simulink model "Aileron_AFTC"  (Simulink 8.6)
settings: Solver=FixedStepAuto  StartTime=0.0  StopTime=40  FixedStep=0.01  RelTol=1e-3
libraries: fuzblock x4, simulink x2
settings Model: Creator=Alireza  LastModifiedBy=aabba014
settings SolverCC: ZeroCrossAlgorithm=Adaptive
settings DebuggingCC: FcnCallInpInsideContextMsg=UseLocalSettings

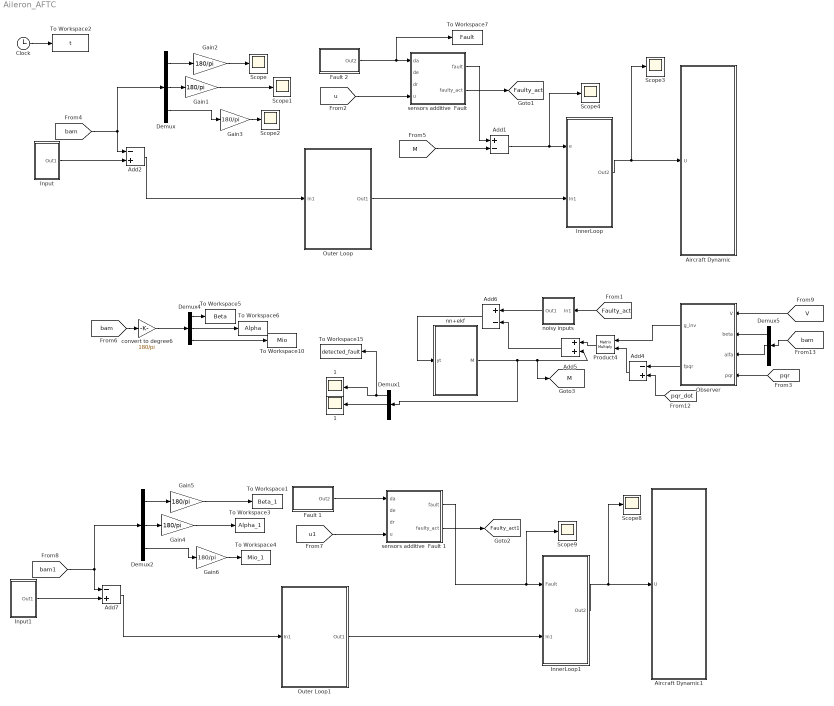
== system Aileron_AFTC ==
  "      1" : Scope
  "     1" : Scope
  Add1 : Sum  Inputs=+-
  Add2 : Sum  Inputs=-+
  Add4 : Sum  Inputs=-+
  Add5 : Sum
  Add6 : Sum  Inputs=+-  OutDataTypeStr=Inherit: Same as accumulator
  Add7 : Sum  Inputs=-+
  Aircraft Dynamic : Subsystem
  Aircraft Dynamic1 : Subsystem
  Clock : Clock
  Demux{,1..2,4..5} (5 alike) : Demux  Outputs=3
  Fault 1 : Subsystem
  Fault 2 : Subsystem
  Gain{1..6} (6 alike) : Gain  Gain=180/pi
  InnerLoop : Subsystem
  InnerLoop1 : Subsystem
  Input : Subsystem
  Input1 : Subsystem
  Observer : MATLAB Function  TreatAsAtomicUnit=on
  Outer Loop : Subsystem
  Outer Loop1 : Subsystem
  Product4 : Product  Multiplication=Matrix(*)  RndMeth=Zero
  Scope{,1..4,8..9} (7 alike) : Scope
  To Workspace1 : ToWorkspace  VariableName=Beta_1  SampleTime=-1
  To Workspace10 : ToWorkspace  VariableName=Mio  SampleTime=-1
  To Workspace15 : ToWorkspace  VariableName=detected_fault  SampleTime=-1
  To Workspace2 : ToWorkspace  VariableName=t  SampleTime=-1
  To Workspace3 : ToWorkspace  VariableName=Alpha_1  SampleTime=-1
  To Workspace4 : ToWorkspace  VariableName=Mio_1  SampleTime=-1
  To Workspace5 : ToWorkspace  VariableName=Beta  SampleTime=-1
  To Workspace6 : ToWorkspace  VariableName=Alpha  SampleTime=-1
  To Workspace7 : ToWorkspace  VariableName=Fault  SampleTime=-1
  convert to degree6 : Gain  Gain=180/pi
  nn+ekf : Subsystem
  noisy inputs : Subsystem
  "sensors additive  Fault " : MATLAB Function  TreatAsAtomicUnit=on
  sensors additive  Fault 1 : MATLAB Function  TreatAsAtomicUnit=on
  tag scope: Faulty_act1=global, Faulty_act=global, M=global
  wires:
  [bam] -> Add2/1, Demux/1
  Input/1(Out1) -> Add2/2
  Outer Loop/1(Out1) -> InnerLoop/2(In1)
  InnerLoop/1(Out2) -> Scope3/1, Aircraft Dynamic/1(U)
  Add2/1 -> Outer Loop/1(In1)
  Demux/1 -> Gain2/1
  Demux/2 -> Gain1/1
  Demux/3 -> Gain3/1
  Gain2/1 -> Scope/1
  Gain1/1 -> Scope1/1
  Gain3/1 -> Scope2/1
  [u] -> "sensors additive  Fault "/4(u)
  "sensors additive  Fault "/2(faulty_act) -> [Faulty_act]
  Add1/1 -> InnerLoop/1(e), Scope4/1
  "sensors additive  Fault "/1(fault) -> Add1/1
  Clock/1 -> To Workspace2/1
  Add5/1 -> Add6/2
  Add6/1 -> nn+ekf/1(yt)
  [bam] -> convert to degree6/1
  [V] -> Observer/1(V)
  [bam] -> Demux5/1
  nn+ekf/1(M) -> Add5/2, [M], Demux1/1
  Demux1/1 -> "     1"/1, To Workspace15/1
  Demux1/2 -> "      1"/1
  convert to degree6/1 -> Demux4/1
  [Faulty_act] -> noisy inputs/1(In1)
  Demux4/1 -> To Workspace5/1
  Demux4/2 -> To Workspace6/1
  Demux4/3 -> To Workspace10/1
  Demux5/1 -> Observer/2(beta)
  Demux5/2 -> Observer/3(alfa)
  [pqr] -> Observer/4(pqr)
  Observer/2(fpqr) -> Add4/1
  [pqr_dot] -> Add4/2
  Add4/1 -> Product4/2
  Observer/1(g_inv) -> Product4/1
  Product4/1 -> Add5/1
  noisy inputs/1(Out1) -> Add6/1
  [M] -> Add1/2
  [bam1] -> Add7/1, Demux2/1
  Input1/1(Out1) -> Add7/2
  Outer Loop1/1(Out1) -> InnerLoop1/2(In1)
  InnerLoop1/1(Out2) -> Aircraft Dynamic1/1(U), Scope8/1
  Add7/1 -> Outer Loop1/1(In1)
  Demux2/1 -> Gain5/1
  Demux2/2 -> Gain4/1
  Demux2/3 -> Gain6/1
  Gain5/1 -> To Workspace1/1
  Gain4/1 -> To Workspace3/1
  [u1] -> sensors additive  Fault 1/4(u)
  sensors additive  Fault 1/2(faulty_act) -> [Faulty_act1]
  sensors additive  Fault 1/1(fault) -> InnerLoop1/1(Fault), Scope9/1
  Gain6/1 -> To Workspace4/1
  Fault 2/1(Out2) -> "sensors additive  Fault "/1(da), To Workspace7/1
  Fault 1/1(Out2) -> sensors additive  Fault 1/1(da)

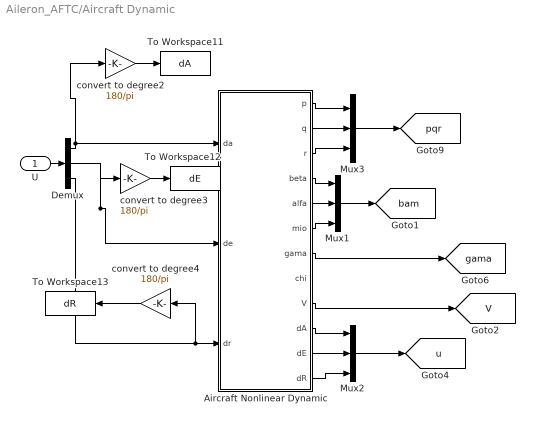
== system Aileron_AFTC/Aircraft Dynamic ==
  U : Inport
  Aircraft Nonlinear Dynamic : Subsystem
  Demux : Demux  Outputs=3
  Mux1 : Mux  Inputs=3
  Mux2 : Mux  Inputs=3
  Mux3 : Mux  Inputs=3
  To Workspace11 : ToWorkspace  VariableName=dA  SampleTime=-1
  To Workspace12 : ToWorkspace  VariableName=dE  SampleTime=-1
  To Workspace13 : ToWorkspace  VariableName=dR  SampleTime=-1
  convert to degree2 : Gain  Gain=180/pi
  convert to degree3 : Gain  Gain=180/pi
  convert to degree4 : Gain  Gain=180/pi
  tag scope: V=global, bam=global, gama=global, pqr=global, u=global
  wires:
  Aircraft Nonlinear Dynamic/4(beta) -> Mux1/1
  Aircraft Nonlinear Dynamic/5(alfa) -> Mux1/2
  Aircraft Nonlinear Dynamic/6(mio) -> Mux1/3
  Mux1/1 -> [bam]
  Aircraft Nonlinear Dynamic/9(V) -> [V]
  Aircraft Nonlinear Dynamic/7(gama) -> [gama]
  Aircraft Nonlinear Dynamic/1(p) -> Mux3/1
  Aircraft Nonlinear Dynamic/2(q) -> Mux3/2
  Aircraft Nonlinear Dynamic/3(r) -> Mux3/3
  Mux3/1 -> [pqr]
  Aircraft Nonlinear Dynamic/10(dA) -> Mux2/1
  Aircraft Nonlinear Dynamic/11(dE) -> Mux2/2
  Aircraft Nonlinear Dynamic/12(dR) -> Mux2/3
  Mux2/1 -> [u]
  convert to degree2/1 -> To Workspace11/1
  convert to degree3/1 -> To Workspace12/1
  Demux/2 -> convert to degree3/1, Aircraft Nonlinear Dynamic/2(de)
  Demux/3 -> Aircraft Nonlinear Dynamic/3(dr), convert to degree4/1
  convert to degree4/1 -> To Workspace13/1
  U/1 -> Demux/1
  Demux/1 -> convert to degree2/1, Aircraft Nonlinear Dynamic/1(da)

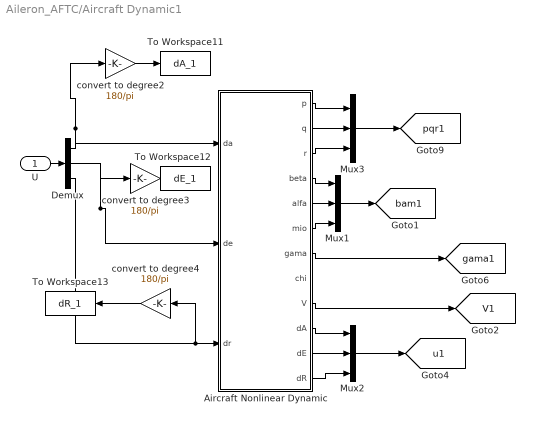
== system Aileron_AFTC/Aircraft Dynamic1 ==
  U : Inport
  Aircraft Nonlinear Dynamic : Subsystem
  Demux : Demux  Outputs=3
  Mux1 : Mux  Inputs=3
  Mux2 : Mux  Inputs=3
  Mux3 : Mux  Inputs=3
  To Workspace11 : ToWorkspace  VariableName=dA_1  SampleTime=-1
  To Workspace12 : ToWorkspace  VariableName=dE_1  SampleTime=-1
  To Workspace13 : ToWorkspace  VariableName=dR_1  SampleTime=-1
  convert to degree2 : Gain  Gain=180/pi
  convert to degree3 : Gain  Gain=180/pi
  convert to degree4 : Gain  Gain=180/pi
  tag scope: V1=global, bam1=global, gama1=global, pqr1=global, u1=global
  wires:
  Aircraft Nonlinear Dynamic/4(beta) -> Mux1/1
  Aircraft Nonlinear Dynamic/5(alfa) -> Mux1/2
  Aircraft Nonlinear Dynamic/6(mio) -> Mux1/3
  Mux1/1 -> [bam1]
  Aircraft Nonlinear Dynamic/9(V) -> [V1]
  Aircraft Nonlinear Dynamic/7(gama) -> [gama1]
  Aircraft Nonlinear Dynamic/1(p) -> Mux3/1
  Aircraft Nonlinear Dynamic/2(q) -> Mux3/2
  Aircraft Nonlinear Dynamic/3(r) -> Mux3/3
  Mux3/1 -> [pqr1]
  Aircraft Nonlinear Dynamic/10(dA) -> Mux2/1
  Aircraft Nonlinear Dynamic/11(dE) -> Mux2/2
  Aircraft Nonlinear Dynamic/12(dR) -> Mux2/3
  Mux2/1 -> [u1]
  convert to degree2/1 -> To Workspace11/1
  convert to degree3/1 -> To Workspace12/1
  Demux/2 -> convert to degree3/1, Aircraft Nonlinear Dynamic/2(de)
  Demux/3 -> Aircraft Nonlinear Dynamic/3(dr), convert to degree4/1
  convert to degree4/1 -> To Workspace13/1
  U/1 -> Demux/1
  Demux/1 -> convert to degree2/1, Aircraft Nonlinear Dynamic/1(da)

== system Aileron_AFTC/Fault 1 ==
  Add13 : Sum  Inputs=+-
  Ramp : simulink/Sources/Ramp  slope=1  start=0  X0=0
  Triangular MF : fuzblock/Membership  Functions/Triangular MF  a=3  b=7  c=11
  Triangular MF1 : fuzblock/Membership  Functions/Triangular MF  a=11  b=15  c=19
  Out2 : Outport
  wires:
  Ramp/1 -> Triangular MF/1, Triangular MF1/1
  Triangular MF/1 -> Add13/1
  Add13/1 -> Out2/1

== system Aileron_AFTC/Fault 2 ==
  Add13 : Sum  Inputs=+-
  Ramp : simulink/Sources/Ramp  slope=1  start=0  X0=0
  Triangular MF : fuzblock/Membership  Functions/Triangular MF  a=3  b=7  c=11
  Triangular MF1 : fuzblock/Membership  Functions/Triangular MF  a=11  b=15  c=19
  Out2 : Outport
  wires:
  Ramp/1 -> Triangular MF/1, Triangular MF1/1
  Triangular MF/1 -> Add13/1
  Add13/1 -> Out2/1

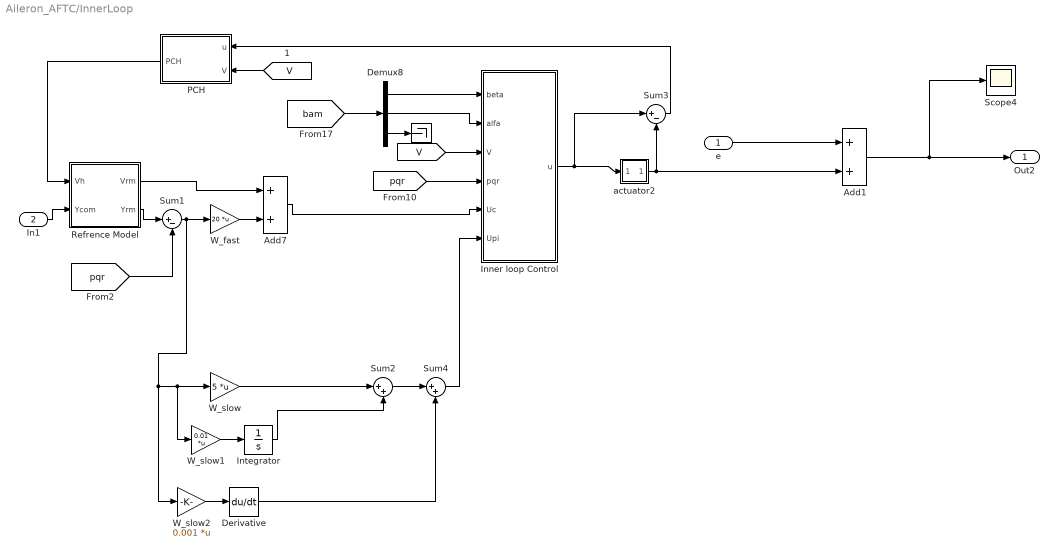
== system Aileron_AFTC/InnerLoop ==
  e : Inport
  In1 : Inport  Port=2
  "  " : Terminator
  Add1 : Sum
  Add7 : Sum
  Demux8 : Demux  Outputs=3
  Derivative : Derivative
  Inner loop Control : MATLAB Function  TreatAsAtomicUnit=on
  Integrator : Integrator
  PCH : MATLAB Function  TreatAsAtomicUnit=on
  Refrence Model : Subsystem
  Scope4 : Scope
  Sum1 : Sum  Inputs=|+-
  Sum2 : Sum  Inputs=|++
  Sum3 : Sum  Inputs=|+-
  Sum4 : Sum  Inputs=|++
  W_fast : Gain  Gain=20  Multiplication=Matrix(K*u)
  W_slow : Gain  Gain=5  Multiplication=Matrix(K*u)
  W_slow1 : Gain  Gain=0.01  Multiplication=Matrix(K*u)
  W_slow2 : Gain  Gain=0.001  Multiplication=Matrix(K*u)
  actuator2 : Subsystem
  Out2 : Outport
  wires:
  [V] -> Inner loop Control/3(V)
  [bam] -> Demux8/1
  Demux8/1 -> Inner loop Control/1(beta)
  Demux8/2 -> Inner loop Control/2(alfa)
  Demux8/3 -> "  "/1
  [pqr] -> Inner loop Control/4(pqr)
  [pqr] -> Sum1/2
  Sum1/1 -> W_fast/1, W_slow1/1, W_slow/1, W_slow2/1
  Add7/1 -> Inner loop Control/5(Uc)
  e/1 -> Add1/1
  [V] -> PCH/2(V)
  W_fast/1 -> Add7/2
  In1/1 -> Refrence Model/2(Ycom)
  Refrence Model/1(Vrm) -> Add7/1
  PCH/1(PCH) -> Refrence Model/1(Vh)
  W_slow/1 -> Sum2/1
  W_slow1/1 -> Integrator/1
  Integrator/1 -> Sum2/2
  Refrence Model/2(Yrm) -> Sum1/1
  W_slow2/1 -> Derivative/1
  Sum2/1 -> Sum4/1
  Derivative/1 -> Sum4/2
  Add1/1 -> Out2/1, Scope4/1
  Inner loop Control/1(u) -> Sum3/1, actuator2/1(In1)
  actuator2/1(Out1) -> Sum3/2, Add1/2
  Sum3/1 -> PCH/1(u)
  Sum4/1 -> Inner loop Control/6(Upi)

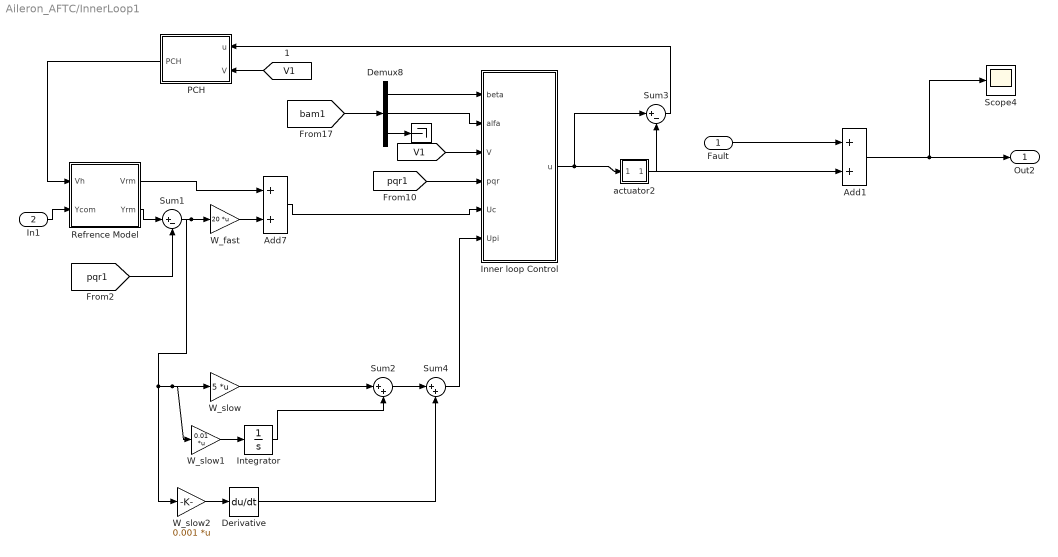
== system Aileron_AFTC/InnerLoop1 ==
  Fault : Inport
  In1 : Inport  Port=2
  "  " : Terminator
  Add1 : Sum
  Add7 : Sum
  Demux8 : Demux  Outputs=3
  Derivative : Derivative
  Inner loop Control : MATLAB Function  TreatAsAtomicUnit=on
  Integrator : Integrator
  PCH : MATLAB Function  TreatAsAtomicUnit=on
  Refrence Model : Subsystem
  Scope4 : Scope
  Sum1 : Sum  Inputs=|+-
  Sum2 : Sum  Inputs=|++
  Sum3 : Sum  Inputs=|+-
  Sum4 : Sum  Inputs=|++
  W_fast : Gain  Gain=20  Multiplication=Matrix(K*u)
  W_slow : Gain  Gain=5  Multiplication=Matrix(K*u)
  W_slow1 : Gain  Gain=0.01  Multiplication=Matrix(K*u)
  W_slow2 : Gain  Gain=0.001  Multiplication=Matrix(K*u)
  actuator2 : Subsystem
  Out2 : Outport
  wires:
  [V1] -> Inner loop Control/3(V)
  [bam1] -> Demux8/1
  Demux8/1 -> Inner loop Control/1(beta)
  Demux8/2 -> Inner loop Control/2(alfa)
  Demux8/3 -> "  "/1
  [pqr1] -> Inner loop Control/4(pqr)
  [pqr1] -> Sum1/2
  Sum1/1 -> W_fast/1, W_slow1/1, W_slow/1, W_slow2/1
  Add7/1 -> Inner loop Control/5(Uc)
  Fault/1 -> Add1/1
  [V1] -> PCH/2(V)
  W_fast/1 -> Add7/2
  In1/1 -> Refrence Model/2(Ycom)
  Refrence Model/1(Vrm) -> Add7/1
  PCH/1(PCH) -> Refrence Model/1(Vh)
  W_slow/1 -> Sum2/1
  W_slow1/1 -> Integrator/1
  Integrator/1 -> Sum2/2
  Refrence Model/2(Yrm) -> Sum1/1
  W_slow2/1 -> Derivative/1
  Sum2/1 -> Sum4/1
  Derivative/1 -> Sum4/2
  Add1/1 -> Out2/1, Scope4/1
  Inner loop Control/1(u) -> Sum3/1, actuator2/1(In1)
  actuator2/1(Out1) -> Sum3/2, Add1/2
  Sum3/1 -> PCH/1(u)
  Sum4/1 -> Inner loop Control/6(Upi)

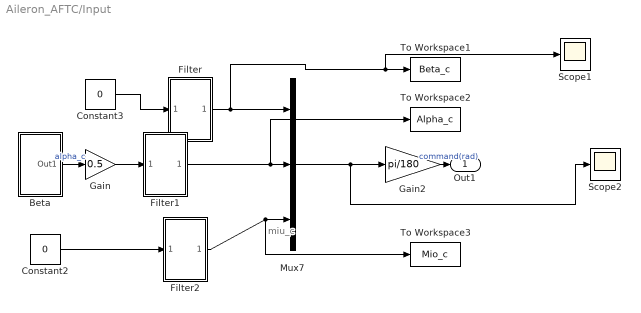
== system Aileron_AFTC/Input ==
  note: miu_c
  Beta : Subsystem
  Constant2 : Constant  Value=0
  Constant3 : Constant  Value=0
  Filter : Subsystem
  Filter1 : Subsystem
  Filter2 : Subsystem
  Gain : Gain  Gain=0.5
  Gain2 : Gain  Gain=pi/180
  Mux7 : Mux  Inputs=3
  Scope1 : Scope
  Scope2 : Scope
  To Workspace1 : ToWorkspace  VariableName=Beta_c  SampleTime=-1
  To Workspace2 : ToWorkspace  VariableName=Alpha_c  SampleTime=-1
  To Workspace3 : ToWorkspace  VariableName=Mio_c  SampleTime=-1
  Out1 : Outport
  wires:
  Beta/1(Out1) -> Gain/1  "alpha_c"
  Constant2/1 -> Filter2/1(In1)
  Mux7/1 -> Gain2/1, Scope2/1
  Gain2/1 -> Out1/1  "command(rad)"
  Filter/1(Out1) -> Mux7/1, To Workspace1/1, Scope1/1
  Filter1/1(Out1) -> Mux7/2, To Workspace2/1
  Filter2/1(Out1) -> Mux7/3, To Workspace3/1
  Constant3/1 -> Filter/1(In1)
  Gain/1 -> Filter1/1(In1)

== system Aileron_AFTC/Input1 ==
  note: miu_c
  Beta : Subsystem
  Constant2 : Constant  Value=0
  Constant3 : Constant  Value=0
  Filter : Subsystem
  Filter1 : Subsystem
  Filter2 : Subsystem
  Gain : Gain  Gain=0.5
  Gain2 : Gain  Gain=pi/180
  Mux7 : Mux  Inputs=3
  Out1 : Outport
  wires:
  Beta/1(Out1) -> Gain/1  "alpha_c"
  Constant2/1 -> Filter2/1(In1)
  Mux7/1 -> Gain2/1
  Gain2/1 -> Out1/1  "command(rad)"
  Filter/1(Out1) -> Mux7/1
  Filter1/1(Out1) -> Mux7/2
  Filter2/1(Out1) -> Mux7/3
  Constant3/1 -> Filter/1(In1)
  Gain/1 -> Filter1/1(In1)

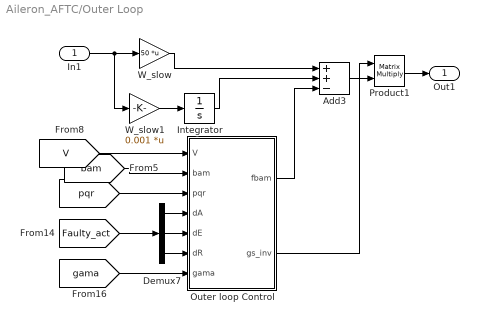
== system Aileron_AFTC/Outer Loop ==
  In1 : Inport
  Add3 : Sum  Inputs=++-
  Demux7 : Demux  Outputs=3
  Integrator : Integrator
  Outer loop Control : MATLAB Function  TreatAsAtomicUnit=on
  Product1 : Product  Multiplication=Matrix(*)  RndMeth=Zero
  W_slow : Gain  Gain=50  Multiplication=Matrix(K*u)
  W_slow1 : Gain  Gain=0.001  Multiplication=Matrix(K*u)
  Out1 : Outport
  wires:
  Outer loop Control/2(gs_inv) -> Product1/1
  Add3/1 -> Product1/2
  [pqr] -> Outer loop Control/3(pqr)
  [bam] -> Outer loop Control/2(bam)
  [V] -> Outer loop Control/1(V)
  [Faulty_act] -> Demux7/1
  Demux7/1 -> Outer loop Control/4(dA)
  Demux7/2 -> Outer loop Control/5(dE)
  Demux7/3 -> Outer loop Control/6(dR)
  [gama] -> Outer loop Control/7(gama)
  In1/1 -> W_slow1/1, W_slow/1
  W_slow/1 -> Add3/1
  W_slow1/1 -> Integrator/1
  Outer loop Control/1(fbam) -> Add3/3
  Integrator/1 -> Add3/2
  Product1/1 -> Out1/1

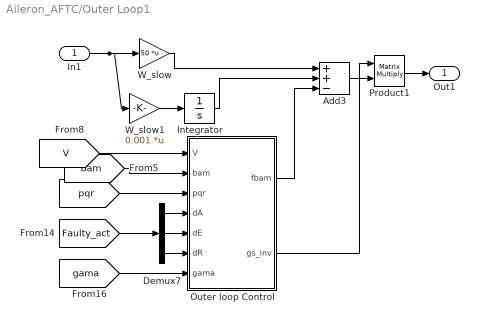
== system Aileron_AFTC/Outer Loop1 ==
  In1 : Inport
  Add3 : Sum  Inputs=++-
  Demux7 : Demux  Outputs=3
  Integrator : Integrator
  Outer loop Control : MATLAB Function  TreatAsAtomicUnit=on
  Product1 : Product  Multiplication=Matrix(*)  RndMeth=Zero
  W_slow : Gain  Gain=50  Multiplication=Matrix(K*u)
  W_slow1 : Gain  Gain=0.001  Multiplication=Matrix(K*u)
  Out1 : Outport
  wires:
  Outer loop Control/2(gs_inv) -> Product1/1
  Add3/1 -> Product1/2
  [pqr] -> Outer loop Control/3(pqr)
  [bam] -> Outer loop Control/2(bam)
  [V] -> Outer loop Control/1(V)
  [Faulty_act] -> Demux7/1
  Demux7/1 -> Outer loop Control/4(dA)
  Demux7/2 -> Outer loop Control/5(dE)
  Demux7/3 -> Outer loop Control/6(dR)
  [gama] -> Outer loop Control/7(gama)
  In1/1 -> W_slow1/1, W_slow/1
  W_slow/1 -> Add3/1
  W_slow1/1 -> Integrator/1
  Outer loop Control/1(fbam) -> Add3/3
  Integrator/1 -> Add3/2
  Product1/1 -> Out1/1

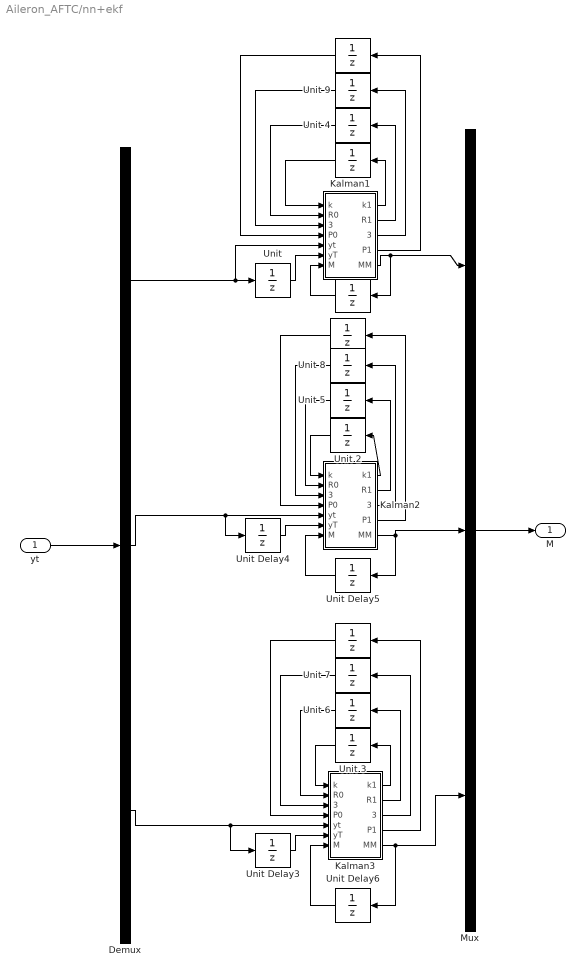
== system Aileron_AFTC/nn+ekf ==
  yt : Inport
  " " : UnitDelay  InitialCondition=1  SampleTime=-1
  "  " : UnitDelay  InitialCondition=5*eye(3)  SampleTime=-1
  "   " : UnitDelay  InitialCondition=5*eye(3)  SampleTime=-1
  "      " : UnitDelay  InitialCondition=.01  SampleTime=-1
  "                " : UnitDelay  InitialCondition=10*eye(3)  SampleTime=-1
  Demux : Demux  Outputs=3
  Kalman1 : MATLAB Function  TreatAsAtomicUnit=on
  Kalman2 : MATLAB Function  TreatAsAtomicUnit=on
  Kalman3 : MATLAB Function  TreatAsAtomicUnit=on
  Mux : Mux  Inputs=3
  "Unit " : UnitDelay  SampleTime=-1
  Unit 2 : UnitDelay  InitialCondition=1  SampleTime=-1
  Unit 3 : UnitDelay  InitialCondition=1  SampleTime=-1
  Unit 4 : UnitDelay  InitialCondition=.00002  SampleTime=-1
  Unit 5 : UnitDelay  InitialCondition=.00002  SampleTime=-1
  Unit 6 : UnitDelay  InitialCondition=.00002  SampleTime=-1
  Unit 7 : UnitDelay  InitialCondition=[1;1;1]  SampleTime=-1
  Unit 8 : UnitDelay  InitialCondition=[1;.5;.5]  SampleTime=-1
  Unit 9 : UnitDelay  InitialCondition=[1;.5;.5]  SampleTime=-1
  Unit Delay3 : UnitDelay  SampleTime=-1
  Unit Delay4 : UnitDelay  SampleTime=-1
  Unit Delay5 : UnitDelay  InitialCondition=.01  SampleTime=-1
  Unit Delay6 : UnitDelay  InitialCondition=.01  SampleTime=-1
  M : Outport
  wires:
  "                "/1 -> Kalman3/4(P0)
  Kalman3/4(P1) -> "                "/1
  "   "/1 -> Kalman2/4(P0)
  Kalman2/4(P1) -> "   "/1
  Unit 8/1 -> Kalman2/3(teta0)
  Kalman2/3(teta1) -> Unit 8/1
  Unit 7/1 -> Kalman3/3(teta0)
  Kalman3/3(teta1) -> Unit 7/1
  Unit 6/1 -> Kalman3/2(R0)
  Kalman3/2(R1) -> Unit 6/1
  Unit 5/1 -> Kalman2/2(R0)
  Kalman2/2(R1) -> Unit 5/1
  Unit 3/1 -> Kalman3/1(k)
  Kalman3/1(k1) -> Unit 3/1
  Unit 2/1 -> Kalman2/1(k)
  Kalman2/1(k1) -> Unit 2/1
  Kalman3/5(MM) -> Unit Delay6/1, Mux/3
  Unit Delay5/1 -> Kalman2/7(M)
  Unit Delay4/1 -> Kalman2/6(yT)
  Unit Delay6/1 -> Kalman3/7(M)
  Unit Delay3/1 -> Kalman3/6(yT)
  Demux/2 -> Kalman2/5(yt), Unit Delay4/1
  Kalman2/5(MM) -> Unit Delay5/1, Mux/2
  Demux/3 -> Kalman3/5(yt), Unit Delay3/1
  Mux/1 -> M/1
  yt/1 -> Demux/1
  "  "/1 -> Kalman1/4(P0)
  Kalman1/4(P1) -> "  "/1
  Unit 9/1 -> Kalman1/3(teta0)
  Kalman1/3(teta1) -> Unit 9/1
  Unit 4/1 -> Kalman1/2(R0)
  Kalman1/2(R1) -> Unit 4/1
  " "/1 -> Kalman1/1(k)
  Kalman1/1(k1) -> " "/1
  "      "/1 -> Kalman1/7(M)
  "Unit "/1 -> Kalman1/6(yT)
  Demux/1 -> Kalman1/5(yt), "Unit "/1
  Kalman1/5(MM) -> "      "/1, Mux/1

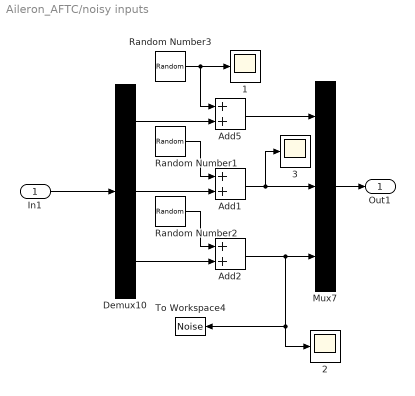
== system Aileron_AFTC/noisy inputs ==
  In1 : Inport
  "     1" : Scope
  "     2" : Scope
  "     3" : Scope
  Add1 : Sum
  Add2 : Sum
  Add5 : Sum
  Demux10 : Demux  Outputs=3
  Mux7 : Mux  Inputs=3
  Random Number1 : RandomNumber  Variance=(0.25*pi/180)^2  Seed=18
  Random Number2 : RandomNumber  Variance=(0.25*pi/180)^2  Seed=40
  Random Number3 : RandomNumber  Variance=(0.25*pi/180)^2  Seed=68
  To Workspace4 : ToWorkspace  VariableName=Noise  SampleTime=-1
  Out1 : Outport
  wires:
  In1/1 -> Demux10/1
  Mux7/1 -> Out1/1
  Random Number3/1 -> Add5/1, "     1"/1
  Demux10/1 -> Add5/2
  Add5/1 -> Mux7/1
  Random Number1/1 -> Add1/1
  Demux10/2 -> Add1/2
  Add1/1 -> Mux7/2, "     3"/1
  Random Number2/1 -> Add2/1
  Demux10/3 -> Add2/2
  Add2/1 -> Mux7/3, "     2"/1, To Workspace4/1

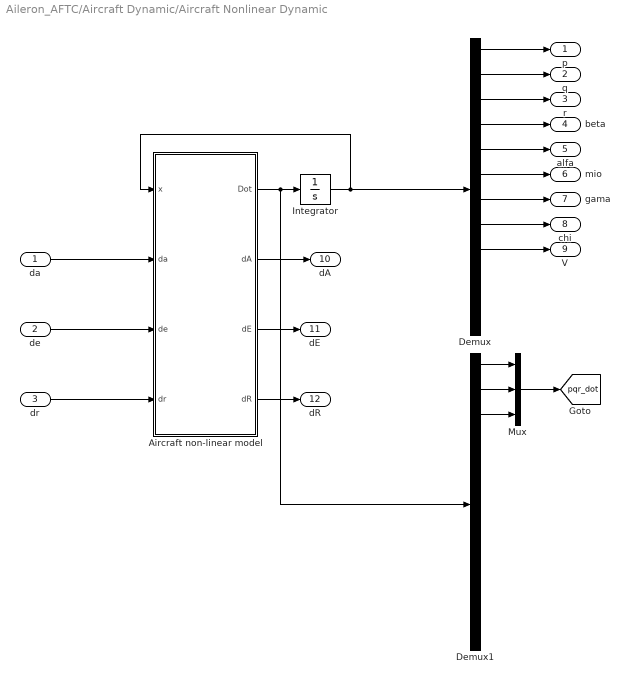
== system Aileron_AFTC/Aircraft Dynamic/Aircraft Nonlinear Dynamic ==
  da : Inport
  de : Inport  Port=2
  dr : Inport  Port=3
  Aircraft non-linear model : MATLAB Function  TreatAsAtomicUnit=on
  Demux : Demux  Outputs=12
  Demux1 : Demux  Outputs=12
  Integrator : Integrator  InitialCondition=[0;0;0;0;0;0;0;0;140;0;2.5*pi/180;0]
  Mux : Mux  Inputs=3
  p : Outport
  q : Outport  Port=2
  r : Outport  Port=3
  beta : Outport  Port=4
  alfa : Outport  Port=5
  mio : Outport  Port=6
  gama : Outport  Port=7
  chi : Outport  Port=8
  V : Outport  Port=9
  dA : Outport  Port=10
  dE : Outport  Port=11
  dR : Outport  Port=12
  tag scope: pqr_dot=global
  wires:
  Aircraft non-linear model/1(Dot) -> Integrator/1, Demux1/1
  Integrator/1 -> Aircraft non-linear model/1(x), Demux/1
  Demux/1 -> p/1
  Demux/2 -> q/1
  Demux/3 -> r/1
  Demux/4 -> beta/1
  Demux/5 -> alfa/1
  Demux/6 -> mio/1
  Demux/7 -> gama/1
  Demux/8 -> chi/1
  Demux/9 -> V/1
  da/1 -> Aircraft non-linear model/2(da)
  de/1 -> Aircraft non-linear model/3(de)
  dr/1 -> Aircraft non-linear model/4(dr)
  Aircraft non-linear model/4(dR) -> dR/1
  Aircraft non-linear model/3(dE) -> dE/1
  Aircraft non-linear model/2(dA) -> dA/1
  Demux1/1 -> Mux/1
  Demux1/2 -> Mux/2
  Demux1/3 -> Mux/3
  Mux/1 -> [pqr_dot]

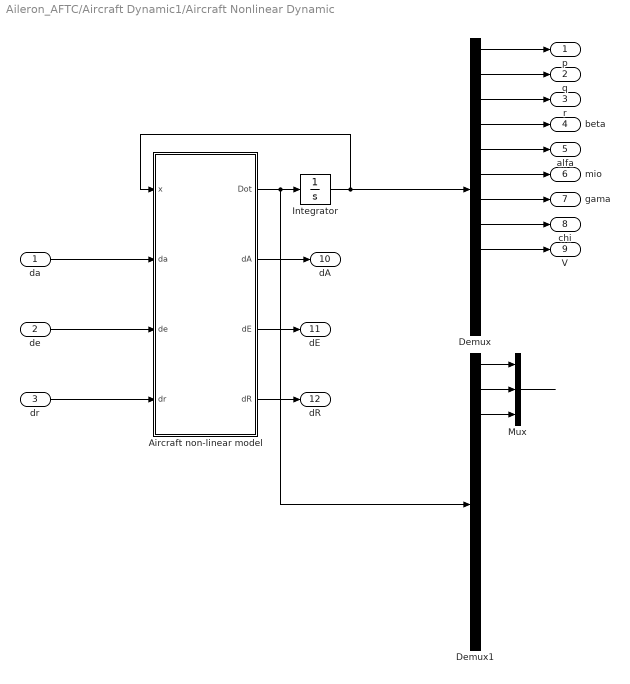
== system Aileron_AFTC/Aircraft Dynamic1/Aircraft Nonlinear Dynamic ==
  da : Inport
  de : Inport  Port=2
  dr : Inport  Port=3
  Aircraft non-linear model : MATLAB Function  TreatAsAtomicUnit=on
  Demux : Demux  Outputs=12
  Demux1 : Demux  Outputs=12
  Integrator : Integrator  InitialCondition=[0;0;0;0;0;0;0;0;140;0;2.5*pi/180;0]
  Mux : Mux  Inputs=3
  p : Outport
  q : Outport  Port=2
  r : Outport  Port=3
  beta : Outport  Port=4
  alfa : Outport  Port=5
  mio : Outport  Port=6
  gama : Outport  Port=7
  chi : Outport  Port=8
  V : Outport  Port=9
  dA : Outport  Port=10
  dE : Outport  Port=11
  dR : Outport  Port=12
  wires:
  Aircraft non-linear model/1(Dot) -> Integrator/1, Demux1/1
  Integrator/1 -> Aircraft non-linear model/1(x), Demux/1
  Demux/1 -> p/1
  Demux/2 -> q/1
  Demux/3 -> r/1
  Demux/4 -> beta/1
  Demux/5 -> alfa/1
  Demux/6 -> mio/1
  Demux/7 -> gama/1
  Demux/8 -> chi/1
  Demux/9 -> V/1
  da/1 -> Aircraft non-linear model/2(da)
  de/1 -> Aircraft non-linear model/3(de)
  dr/1 -> Aircraft non-linear model/4(dr)
  Aircraft non-linear model/4(dR) -> dR/1
  Aircraft non-linear model/3(dE) -> dE/1
  Aircraft non-linear model/2(dA) -> dA/1
  Demux1/1 -> Mux/1
  Demux1/2 -> Mux/2
  Demux1/3 -> Mux/3
  Mux/1 -> ?

== system Aileron_AFTC/InnerLoop/Refrence Model ==
  Vh : Inport
  Ycom : Inport  Port=2
  Add : Sum  Inputs=-+
  Gain : Gain  Gain=100
  Integrator : Integrator  UpperSaturationLimit=3  LowerSaturationLimit=-3
  Sum : Sum  Inputs=|+-
  lat_sat : Saturate  UpperLimit=0.20  LowerLimit=-0.20
  Vrm : Outport
  Yrm : Outport  Port=2
  wires:
  lat_sat/1 -> Sum/1
  Sum/1 -> Gain/1
  Integrator/1 -> Sum/2, Yrm/1
  Ycom/1 -> lat_sat/1
  Gain/1 -> Add/2, Vrm/1
  Vh/1 -> Add/1
  Add/1 -> Integrator/1

== system Aileron_AFTC/InnerLoop/actuator2 ==
  In1 : Inport
  Gain2 : Gain  Gain=20
  Integrator1 : Integrator  InitialCondition=[0;0;0]  UpperSaturationLimit=1.5  LowerSaturationLimit=-1.5
  Saturation : Saturate  UpperLimit=2  LowerLimit=-2
  Sum : Sum  Inputs=|+-
  Out1 : Outport
  wires:
  Sum/1 -> Gain2/1
  In1/1 -> Saturation/1
  Integrator1/1 -> Out1/1, Sum/2
  Gain2/1 -> Integrator1/1
  Saturation/1 -> Sum/1

== system Aileron_AFTC/InnerLoop1/Refrence Model ==
  Vh : Inport
  Ycom : Inport  Port=2
  Add : Sum  Inputs=-+
  Gain : Gain  Gain=100
  Integrator : Integrator  UpperSaturationLimit=3  LowerSaturationLimit=-3
  Sum : Sum  Inputs=|+-
  lat_sat : Saturate  UpperLimit=0.20  LowerLimit=-0.20
  Vrm : Outport
  Yrm : Outport  Port=2
  wires:
  lat_sat/1 -> Sum/1
  Sum/1 -> Gain/1
  Integrator/1 -> Sum/2, Yrm/1
  Ycom/1 -> lat_sat/1
  Gain/1 -> Add/2, Vrm/1
  Vh/1 -> Add/1
  Add/1 -> Integrator/1

== system Aileron_AFTC/InnerLoop1/actuator2 ==
  In1 : Inport
  Gain2 : Gain  Gain=20
  Integrator1 : Integrator  InitialCondition=[0;0;0]  UpperSaturationLimit=1.5  LowerSaturationLimit=-1.5
  Saturation : Saturate  UpperLimit=2  LowerLimit=-2
  Sum : Sum  Inputs=|+-
  Out1 : Outport
  wires:
  Sum/1 -> Gain2/1
  In1/1 -> Saturation/1
  Integrator1/1 -> Out1/1, Sum/2
  Gain2/1 -> Integrator1/1
  Saturation/1 -> Sum/1

== system Aileron_AFTC/Input/Beta ==
  B2 : Step  Time=4  After=60  SampleTime=0
  B3 : Step  Time=14  After=60  SampleTime=0
  Sum2 : Sum  Inputs=|+-
  Out1 : Outport
  wires:
  B2/1 -> Sum2/1
  Sum2/1 -> Out1/1
  B3/1 -> Sum2/2

== system Aileron_AFTC/Input/Filter ==
  In1 : Inport
  Transfer Fcn : TransferFcn  Denominator=[1 1]
  Transfer Fcn1 : TransferFcn  Denominator=[1 1]
  filter4 : Subsystem
  Out1 : Outport
  wires:
  filter4/1(Out) -> Transfer Fcn/1
  Transfer Fcn/1 -> Transfer Fcn1/1
  Transfer Fcn1/1 -> Out1/1
  In1/1 -> filter4/1(In)

== system Aileron_AFTC/Input/Filter1 ==
  In1 : Inport
  Transfer Fcn : TransferFcn  Denominator=[1 1]
  Transfer Fcn1 : TransferFcn  Denominator=[1 1]
  filter4 : Subsystem
  Out1 : Outport
  wires:
  In1/1 -> filter4/1(In)
  Transfer Fcn1/1 -> Out1/1
  Transfer Fcn/1 -> Transfer Fcn1/1
  filter4/1(Out) -> Transfer Fcn/1

== system Aileron_AFTC/Input/Filter2 ==
  In1 : Inport
  Transfer Fcn : TransferFcn  Denominator=[1 1]
  Transfer Fcn1 : TransferFcn  Denominator=[1 1]
  filter4 : Subsystem
  Out1 : Outport
  wires:
  filter4/1(Out) -> Transfer Fcn/1
  Transfer Fcn/1 -> Transfer Fcn1/1
  Transfer Fcn1/1 -> Out1/1
  In1/1 -> filter4/1(In)

== system Aileron_AFTC/Input1/Beta ==
  B2 : Step  Time=4  After=60  SampleTime=0
  B3 : Step  Time=14  After=60  SampleTime=0
  Sum2 : Sum  Inputs=|+-
  Out1 : Outport
  wires:
  B2/1 -> Sum2/1
  Sum2/1 -> Out1/1
  B3/1 -> Sum2/2

== system Aileron_AFTC/Input1/Filter ==
  In1 : Inport
  Transfer Fcn : TransferFcn  Denominator=[1 1]
  Transfer Fcn1 : TransferFcn  Denominator=[1 1]
  filter4 : Subsystem
  Out1 : Outport
  wires:
  filter4/1(Out) -> Transfer Fcn/1
  Transfer Fcn/1 -> Transfer Fcn1/1
  Transfer Fcn1/1 -> Out1/1
  In1/1 -> filter4/1(In)

== system Aileron_AFTC/Input1/Filter1 ==
  In1 : Inport
  Transfer Fcn : TransferFcn  Denominator=[1 1]
  Transfer Fcn1 : TransferFcn  Denominator=[1 1]
  filter4 : Subsystem
  Out1 : Outport
  wires:
  In1/1 -> filter4/1(In)
  Transfer Fcn1/1 -> Out1/1
  Transfer Fcn/1 -> Transfer Fcn1/1
  filter4/1(Out) -> Transfer Fcn/1

== system Aileron_AFTC/Input1/Filter2 ==
  In1 : Inport
  Transfer Fcn : TransferFcn  Denominator=[1 1]
  Transfer Fcn1 : TransferFcn  Denominator=[1 1]
  filter4 : Subsystem
  Out1 : Outport
  wires:
  filter4/1(Out) -> Transfer Fcn/1
  Transfer Fcn/1 -> Transfer Fcn1/1
  Transfer Fcn1/1 -> Out1/1
  In1/1 -> filter4/1(In)

== system Aileron_AFTC/Input/Filter/filter4 ==
  In : Inport
  Gain1 : Gain  Gain=25
  Gain2 : Gain  Gain=20
  Gain4 : Gain  Gain=25
  Integrator10 : Integrator
  Integrator8 : Integrator
  Sum5 : Sum  Inputs=||+--
  Out : Outport
  wires:
  Sum5/1 -> Integrator8/1
  Integrator8/1 -> Integrator10/1, Gain2/1
  Gain2/1 -> Sum5/3
  Integrator10/1 -> Gain4/1, Out/1
  Gain4/1 -> Sum5/2
  Gain1/1 -> Sum5/1
  In/1 -> Gain1/1

== system Aileron_AFTC/Input/Filter1/filter4 ==
  In : Inport
  Gain1 : Gain  Gain=25
  Gain2 : Gain  Gain=20
  Gain4 : Gain  Gain=25
  Integrator10 : Integrator
  Integrator8 : Integrator
  Sum5 : Sum  Inputs=||+--
  Out : Outport
  wires:
  In/1 -> Gain1/1
  Gain1/1 -> Sum5/1
  Gain4/1 -> Sum5/2
  Integrator10/1 -> Out/1, Gain4/1
  Gain2/1 -> Sum5/3
  Integrator8/1 -> Gain2/1, Integrator10/1
  Sum5/1 -> Integrator8/1

== system Aileron_AFTC/Input/Filter2/filter4 ==
  In : Inport
  Gain1 : Gain  Gain=25
  Gain2 : Gain  Gain=20
  Gain4 : Gain  Gain=25
  Integrator10 : Integrator
  Integrator8 : Integrator
  Sum5 : Sum  Inputs=||+--
  Out : Outport
  wires:
  Sum5/1 -> Integrator8/1
  Integrator8/1 -> Integrator10/1, Gain2/1
  Gain2/1 -> Sum5/3
  Integrator10/1 -> Gain4/1, Out/1
  Gain4/1 -> Sum5/2
  Gain1/1 -> Sum5/1
  In/1 -> Gain1/1

== system Aileron_AFTC/Input1/Filter/filter4 ==
  In : Inport
  Gain1 : Gain  Gain=25
  Gain2 : Gain  Gain=20
  Gain4 : Gain  Gain=25
  Integrator10 : Integrator
  Integrator8 : Integrator
  Sum5 : Sum  Inputs=||+--
  Out : Outport
  wires:
  Sum5/1 -> Integrator8/1
  Integrator8/1 -> Integrator10/1, Gain2/1
  Gain2/1 -> Sum5/3
  Integrator10/1 -> Gain4/1, Out/1
  Gain4/1 -> Sum5/2
  Gain1/1 -> Sum5/1
  In/1 -> Gain1/1

== system Aileron_AFTC/Input1/Filter1/filter4 ==
  In : Inport
  Gain1 : Gain  Gain=25
  Gain2 : Gain  Gain=20
  Gain4 : Gain  Gain=25
  Integrator10 : Integrator
  Integrator8 : Integrator
  Sum5 : Sum  Inputs=||+--
  Out : Outport
  wires:
  In/1 -> Gain1/1
  Gain1/1 -> Sum5/1
  Gain4/1 -> Sum5/2
  Integrator10/1 -> Out/1, Gain4/1
  Gain2/1 -> Sum5/3
  Integrator8/1 -> Gain2/1, Integrator10/1
  Sum5/1 -> Integrator8/1

== system Aileron_AFTC/Input1/Filter2/filter4 ==
  In : Inport
  Gain1 : Gain  Gain=25
  Gain2 : Gain  Gain=20
  Gain4 : Gain  Gain=25
  Integrator10 : Integrator
  Integrator8 : Integrator
  Sum5 : Sum  Inputs=||+--
  Out : Outport
  wires:
  Sum5/1 -> Integrator8/1
  Integrator8/1 -> Integrator10/1, Gain2/1
  Gain2/1 -> Sum5/3
  Integrator10/1 -> Gain4/1, Out/1
  Gain4/1 -> Sum5/2
  Gain1/1 -> Sum5/1
  In/1 -> Gain1/1

== matlab function InnerLoop/Inner loop Control ==
  data: beta input double; alfa input double; u output double; V input double; pqr input double; Uc input double; Upi input double
function u  = fcn(beta,alfa,V,pqr,Uc,Upi)

p=pqr(1);
q=pqr(2);
r=pqr(3);
%====================================
% Equations Of Motion
ro=.4139;%====================================================================================
cbar = 1.164; %======== m ========
c=cbar;
b = 25.83; %======== m ========
Ix = 2405;
Iy = 13987;
Iz = 14496;
Ixz = 909;
s = 27.8; %========= m^2 =======
Q=0.5*ro*V^2;
Clbeta=-0.0008569*180/pi; %per rad
Clp=-0.7417551; %per rad
Clr=0.1887752; %per rad
Cmq=-12.10793; %per rad
CldA=.0037483*180/pi; %per rad
CldR=.0006043*180/pi; %per rad
CmdE=-.0232702*180/pi; %per rad
Cnbeta=.0014660*180/pi; %per rad
Cnp=-0.0591078; %per rad
Cnr=-0.4654417; %per rad
CndA=.0000309*180/pi; %per rad
CndR=-.0010612*180/pi ; %per rad
Cm0= 0.0102;
Cmalfa=-1.31; % =========  1/rad =============
%===============================================
Cm =Cm0+cbar/(2*V)*Cmq*q;
%===============================================
L_aero=Q*s*b*(Clbeta*beta+(Clp*p+Clr*r)*b/(2*V));
M_aero=Q*s*c*(Cm0+Cmalfa*alfa+Cmq*q*c/(2*V));
N_aero=Q*s*b*(Cnbeta*beta+(Cnp*p+Cnr*r)*b/(2*V));

%==============================
f1=(Iz*L_aero+Ixz*N_aero+Ixz*(Ix-Iy+Iz)*p*q+(Iz*(Iy-Iz)-Ixz^2)*q*r)/(Ix*Iz-Ixz^2);
f2=(M_aero+p*r*(Iz-Ix)+Ixz*(r^2-p^2))/Iy;
f3=(Ixz*L_aero+Ix*N_aero+(Ix*(Ix-Iy)+Ixz^2)*p*q-Ixz*(Ix-Iy+Iz)*q*r)/(Ix*Iz-Ixz^2);


%==============================
LdA=(1/(Ix*Iz-Ixz^2))*(Q*s*b)*(Iz*CldA+Ixz*CndA);
LdR=(1/(Ix*Iz-Ixz^2))*(Q*s*b)*(Iz*CldR+Ixz*CndR);
MdE=(1/(Iy))*(Q*s*c)*CmdE;
NdA=(1/(Ix*Iz-Ixz^2))*(Q*s*b)*(Ix*CndA+Ixz*CldA);
NdR=(1/(Ix*Iz-Ixz^2))*(Q*s*b)*(Ix*CndR+Ixz*CldR);
%==============================
f_pqr=[f1;f2;f3];
B=([LdA 0 LdR;0 MdE 0;NdA 0 NdR]);
u=B\(Uc-f_pqr+Upi);

== matlab function Aircraft Dynamic/Aircraft Nonlinear Dynamic/Aircraft non-linear model ==
  data: x input double; da input double; Dot output double; de input double; dr input double; dA output double; dE output double; dR output double
 function [Dot,dA,dE,dR] = fcn(x,da,de,dr)
%====================================
%% States Variable
p = x(1);
q = x(2);
r = x(3);
beta = x(4);
alfa = x(5);
mio = x(6);
gama = x(7);
chi = x(8);
V = x(9);
phi = x(10);
theta = x(11);
psi = x(12);
%====================================
% Equations Of Motion
M = 5000; %=== mass  kg
th=1;
u0=140;%===================== m/s ==================
ro=.0889;%====================================================================================
T = 13000*th*ro/1.225; %======== N ============
cbar = 1.164; %======== m ========
c=cbar;
b = 25.83; %======== m ========
Ix = 2405;
Iy = 13987;
Iz = 14496;
Ixz = 909;
s = 27.8; %========= m^2 =======
CLalfa=6.8; %per rad
CLq = 6.319133; %per rad
CLdE=.0054746*180/pi; %per rad
Q=0.5*ro*V^2;
Cybeta=-0.0073848*180/pi; %per rad
Cyp=0.0367876; %per rad
Cyr=-1.5779230; %per rad
CydR=-.0050774*180/pi; %per rad
CD0=0.0165;
CDdE=.0128281*180/pi; %per rad
CDq=2.580423; %per rad
g = 9.81; %=== m/s^2 =====
Clbeta=-0.0008569*180/pi; %per rad
Clp=-0.7417551; %per rad
Clr=0.1887752; %per rad
Cmq=-12.10793; %per rad
CldA=.0037483*180/pi; %per rad
CldR=.0006043*180/pi; %per rad
CmdE=-.0232702*180/pi; %per rad
Cnbeta=.0014660*180/pi; %per rad
Cnp=-0.0591078; %per rad
Cnr=-0.4654417; %per rad
CndA=.0000309*180/pi; %per rad
CndR=-.0010612*180/pi ; %per rad
CydA=.0001716*180/pi; %per rad
CL0=0.46;
Cm0= 0.0102;
Cmalfa=-1.31; % =========  1/rad =============
dA=da;
dE=de;
dR=dr;
%===============================================
Cm=Cm0+cbar/(2*V)*Cmq*q;
%===============================================
laero=Q*s*b*(Clbeta*beta+(Clp*p+Clr*r)*b/(2*V)+CldA*dA+CldR*dR);
maero=Q*s*c*(Cm0+Cmalfa*alfa+Cmq*q*c/(2*V)+CmdE*dE);
naero=Q*s*b*(Cnbeta*beta+(Cnp*p+Cnr*r)*b/(2*V)+CndA*dA+CndR*dR);
%===============================================
Ybeta=Q*s*Cybeta/M;% (m/s^2)
Yp=Q*s*b*Cyp/(2*M*V);% (m/s)
Yr=Q*s*b*Cyr/(2*M*V);% (m/s)
YdR=Q*s*CydR/M; % (m/s^2)
YdA=Q*s*CydA/M; % (m/s^2)
%================================================
Y=M*(Ybeta*beta+Yp*p+Yr*r+YdR*dR+YdA*dA);
L=Q*s*(CL0+CLalfa*alfa+cbar/(2*V)*CLq*q+CLdE*dE);
D=Q*s*(CD0+cbar/(2*V)*CDq*q+CDdE*abs(dE)/4);
%================================================
pdot=((Iz*laero+Ixz*naero)/(Ix*Iz-Ixz^2))+(Ixz*(Ix-Iy+Iz)*p*q+(Iz*(Iy-Iz)-Ixz^2)*q*r)/(Ix*Iz-Ixz^2);
qdot=(1/Iy)*(maero+p*r*(Iz-Ix)+Ixz*(r^2-p^2));
rdot=((Ixz*laero+Ix*naero)/(Ix*Iz-Ixz^2))+(((Ix*(Ix-Iy)+Ixz^2)*p*q-Ixz*(Ix-Iy+Iz)*q*r)/(Ix*Iz-Ixz^2));
%================================================
betadot=p*sin(alfa)-r*cos(alfa)+((M*g*cos(gama)*sin(mio))+(Y*cos(beta)-T*sin(beta)*cos(alfa)))/(M*V);
alfadot=q-(p*cos(alfa)+r*sin(alfa))*tan(beta)+(-L+M*g*cos(gama)*cos(mio)-T*sin(alfa))/(M*V*cos(beta));
miodot=1/cos(beta)*(p*cos(alfa)+r*sin(alfa))-g/V*tan(beta)*cos(mio)*cos(gama)+(L+T*sin(alfa))/(M*V)*(tan(gama)*sin(mio)+tan(beta))+Y/(M*V)*tan(gama)*cos(mio)*cos(beta);
%================================================
gamadot=((1/(M*V))*(-D*sin(beta)*sin(mio)+L*cos(mio)-M*g*cos(gama)-Y*sin(mio)*cos(beta)))+((T/(M*V))*(sin(mio)*sin(beta)*cos(alfa)+cos(mio)*sin(alfa)));
chidot=((L*sin(mio)+Y*cos(mio)*cos(beta))+T*(sin(mio)*sin(alfa)-cos(mio)*sin(beta)*cos(alfa)))/(M*V*cos(gama));
Vdot=(-D*cos(beta)+Y*sin(beta)-M*g*sin(gama)+T*cos(beta)*cos(alfa))/M;
%================================================
phidot=p+q*sin(phi)*tan(theta)+r*cos(phi)*tan(theta);
thetadot=q*cos(phi)-r*sin(phi);
psidot=(q*sin(phi)+r*cos(phi))/cos(theta);
%================================================
Dot=[pdot;qdot;rdot;betadot;alfadot;miodot;gamadot;chidot;Vdot;phidot;thetadot;psidot];

== matlab function sensors additive  Fault  ==
  data: da input double; de input double; dr input double; fault output double; u input double; faulty_act output double
function [fault,faulty_act] = fcn(da,de,dr,u)
fault=[da;de;dr];
faulty_act=fault+u;

== matlab function Outer Loop/Outer loop Control ==
  data: fbam output double; V input double; gs_inv output double; bam input double; pqr input double; dA input double; dE input double; dR input double; gama input double
function [fbam,gs_inv] = fcn(V,bam,pqr,dA,dE,dR,gama)
beta=bam(1);
alfa=bam(2);
mio=bam(3);
p=pqr(1);
q=pqr(2);
r=pqr(3);
% inputs ////////////////////
M = 5000; %=== mass  kg
th=1;
u0=140;%========================================================================================
ro=.4139;%====================================================================================
T = 13000*th*ro/1.225; %======== N ============
cbar = 1.164; %======== m ========
c=cbar;
b = 25.83; %======== m ========
s = 27.8; %========= m^2 =======
CLalfa=6.8; %per rad
CLq = 6.319133; %per rad
CLdE=.0054746*180/pi; %per rad
CLu=0;
Q=0.5*ro*V^2;
Cybeta=-0.0073848*180/pi; %per rad
Cyp=0.0367876; %per rad
Cyr=-1.5779230; %per rad
CydR=-.0050774*180/pi; %per rad
g = 9.81; %=== m/s^2 =====
CydA=.0001716*180/pi; %per rad
CL0=0.46;
%===============================================
Ybeta=Q*s*Cybeta/M;% (m/s^2)
Yp=Q*s*b*Cyp/(2*M*u0);% (m/s)
Yr=Q*s*b*Cyr/(2*M*u0);% (m/s)
YdR=Q*s*CydR/M; % (m/s^2)
YdA=Q*s*CydA/M; % (m/s^2)
%================================================
Y=M*(Ybeta*beta+Yp*p+Yr*r+YdR*dR+YdA*dA);
L=Q*s*(CL0+cbar/(2*V)*CLq*q+CLdE*dE);
%==============================
f1=(1/(M*V))*(Y*cos(beta)+M*g*sin(gama)*sin(mio)-T*sin(beta)*cos(alfa));
f2=(1/(M*V*cos(beta)))*(-L+M*g*cos(gama)*cos(mio)-T*sin(alfa));
f3=-g/V*tan(beta)*cos(mio)*cos(gama)+(1/(M*V))*((L+T*sin(alfa))*(tan(gama)*sin(mio)+tan(beta))+Y*tan(gama)*cos(mio)*cos(beta));
%==============================
fbam=[f1;f2;f3];
gs_inv=([sin(alfa) 0 -cos(alfa);-tan(beta)*cos(alfa) 1 -tan(beta)*sin(alfa);cos(alfa)/cos(beta) 0 sin(alfa)/cos(beta)])^-1;

== matlab function Observer ==
  data: V input double; beta input double; alfa input double; pqr input double; g_inv output double; fpqr output double
function [g_inv,fpqr]   = fcn(V,beta,alfa,pqr)
p=pqr(1);
q=pqr(2);
r=pqr(3);
% Equations Of Motion
ro=.0889;%====================================================================================
cbar = 1.164; %======== m ========
c=cbar;
b = 25.83; %======== m ========
Ix = 2405;
Iy = 13987;
Iz = 14496;
Ixz = 909;
s = 27.8; %========= m^2 =======
Q=0.5*ro*V^2;
Clbeta=-0.0008569*180/pi; %per rad
Clp=-0.7417551; %per rad
Clr=0.1887752; %per rad
Cmq=-12.10793; %per rad
CldA=.0037483*180/pi; %per rad
CldR=.0006043*180/pi; %per rad
CmdE=-.0232702*180/pi; %per rad
Cnbeta=.0014660*180/pi; %per rad
Cnp=-0.0591078; %per rad
Cnr=-0.4654417; %per rad
CndA=.0000309*180/pi; %per rad
CndR=-.0010612*180/pi ; %per rad
Cm0= 0.0102;
Cmalfa=-1.31; % =========  1/rad =============
%===============================================
Cm =Cm0+cbar/(2*V)*Cmq*q;
%===============================================
laerohat=Q*s*b*(Clbeta*beta+(Clp*p+Clr*r)*b/(2*V));
maerohat=Q*s*c*(Cm0+Cmalfa*alfa+Cmq*q*c/(2*V));
naerohat=Q*s*b*(Cnbeta*beta+(Cnp*p+Cnr*r)*b/(2*V));
%===============================================
f1=(Iz*laerohat+Ixz*naerohat+Ixz*(Ix-Iy+Iz)*p*q+(Iz*(Iy-Iz)-Ixz^2)*q*r)/(Ix*Iz-Ixz^2);
f2=(maerohat+p*r*(Iz-Ix)+Ixz*(r^2-p^2))/Iy;
f3=(Ixz*laerohat+Ix*naerohat+(Ix*(Ix-Iy)+Ixz^2)*p*q-Ixz*(Ix-Iy+Iz)*q*r)/(Ix*Iz-Ixz^2);
%==============================
LdA=(1/(Ix*Iz-Ixz^2))*(Q*s*b)*(Iz*CldA+Ixz*CndA);
LdR=(1/(Ix*Iz-Ixz^2))*(Q*s*b)*(Iz*CldR+Ixz*CndR);
MdE=(1/(Iy))*(Q*s*c)*CmdE;
NdA=(1/(Ix*Iz-Ixz^2))*(Q*s*b)*(Ix*CndA+Ixz*CldA);
NdR=(1/(Ix*Iz-Ixz^2))*(Q*s*b)*(Ix*CndR+Ixz*CldR);
%==============================
fpqr=[f1;f2;f3];
g=[LdA 0 LdR;0 MdE 0;NdA 0 NdR];
g_inv=g^(-1);

== matlab function InnerLoop/PCH ==
  data: u input double; PCH output double; V input double
function PCH= fcn(u,V)


%====================================
% Equations Of Motion
ro=.4139;%====================================================================================
cbar = 1.164; %======== m ========
c=cbar;
b = 25.83; %======== m ========
Ix = 2405;
Iy = 13987;
Iz = 14496;
Ixz = 909;
s = 27.8; %========= m^2 =======
Q=0.5*ro*V^2;
Clbeta=-0.0008569*180/pi; %per rad
Clp=-0.7417551; %per rad
Clr=0.1887752; %per rad
Cmq=-12.10793; %per rad
CldA=.0037483*180/pi; %per rad
CldR=.0006043*180/pi; %per rad
CmdE=-.0232702*180/pi; %per rad
Cnbeta=.0014660*180/pi; %per rad
Cnp=-0.0591078; %per rad
Cnr=-0.4654417; %per rad
CndA=.0000309*180/pi; %per rad
CndR=-.0010612*180/pi ; %per rad
Cm0= 0.0102;
Cmalfa=-1.31; % =========  1/rad =============
%===============================================
LdA=(1/(Ix*Iz-Ixz^2))*(Q*s*b)*(Iz*CldA+Ixz*CndA);
LdR=(1/(Ix*Iz-Ixz^2))*(Q*s*b)*(Iz*CldR+Ixz*CndR);
MdE=(1/(Iy))*(Q*s*c)*CmdE;
NdA=(1/(Ix*Iz-Ixz^2))*(Q*s*b)*(Ix*CndA+Ixz*CldA);
NdR=(1/(Ix*Iz-Ixz^2))*(Q*s*b)*(Ix*CndR+Ixz*CldR);
%==============================
B=([LdA 0 LdR;0 MdE 0;NdA 0 NdR]);
PCH=B*u;

== matlab function Aircraft Dynamic1/Aircraft Nonlinear Dynamic/Aircraft non-linear model ==
  data: x input double; da input double; Dot output double; de input double; dr input double; dA output double; dE output double; dR output double
 function [Dot,dA,dE,dR] = fcn(x,da,de,dr)
%====================================
%% States Variable
p = x(1);
q = x(2);
r = x(3);
beta = x(4);
alfa = x(5);
mio = x(6);
gama = x(7);
chi = x(8);
V = x(9);
phi = x(10);
theta = x(11);
psi = x(12);
%====================================
% Equations Of Motion
M = 5000; %=== mass  kg
th=1;
u0=140;%===================== m/s ==================
ro=.0889;%====================================================================================
T = 13000*th*ro/1.225; %======== N ============
cbar = 1.164; %======== m ========
c=cbar;
b = 25.83; %======== m ========
Ix = 2405;
Iy = 13987;
Iz = 14496;
Ixz = 909;
s = 27.8; %========= m^2 =======
CLalfa=6.8; %per rad
CLq = 6.319133; %per rad
CLdE=.0054746*180/pi; %per rad
Q=0.5*ro*V^2;
Cybeta=-0.0073848*180/pi; %per rad
Cyp=0.0367876; %per rad
Cyr=-1.5779230; %per rad
CydR=-.0050774*180/pi; %per rad
CD0=0.0165;
CDdE=.0128281*180/pi; %per rad
CDq=2.580423; %per rad
g = 9.81; %=== m/s^2 =====
Clbeta=-0.0008569*180/pi; %per rad
Clp=-0.7417551; %per rad
Clr=0.1887752; %per rad
Cmq=-12.10793; %per rad
CldA=.0037483*180/pi; %per rad
CldR=.0006043*180/pi; %per rad
CmdE=-.0232702*180/pi; %per rad
Cnbeta=.0014660*180/pi; %per rad
Cnp=-0.0591078; %per rad
Cnr=-0.4654417; %per rad
CndA=.0000309*180/pi; %per rad
CndR=-.0010612*180/pi ; %per rad
CydA=.0001716*180/pi; %per rad
CL0=0.46;
Cm0= 0.0102;
Cmalfa=-1.31; % =========  1/rad =============
dA=da;
dE=de;
dR=dr;
%===============================================
Cm=Cm0+cbar/(2*V)*Cmq*q;
%===============================================
laero=Q*s*b*(Clbeta*beta+(Clp*p+Clr*r)*b/(2*V)+CldA*dA+CldR*dR);
maero=Q*s*c*(Cm0+Cmalfa*alfa+Cmq*q*c/(2*V)+CmdE*dE);
naero=Q*s*b*(Cnbeta*beta+(Cnp*p+Cnr*r)*b/(2*V)+CndA*dA+CndR*dR);
%===============================================
Ybeta=Q*s*Cybeta/M;% (m/s^2)
Yp=Q*s*b*Cyp/(2*M*V);% (m/s)
Yr=Q*s*b*Cyr/(2*M*V);% (m/s)
YdR=Q*s*CydR/M; % (m/s^2)
YdA=Q*s*CydA/M; % (m/s^2)
%================================================
Y=M*(Ybeta*beta+Yp*p+Yr*r+YdR*dR+YdA*dA);
L=Q*s*(CL0+CLalfa*alfa+cbar/(2*V)*CLq*q+CLdE*dE);
D=Q*s*(CD0+cbar/(2*V)*CDq*q+CDdE*abs(dE)/4);
%================================================
pdot=((Iz*laero+Ixz*naero)/(Ix*Iz-Ixz^2))+(Ixz*(Ix-Iy+Iz)*p*q+(Iz*(Iy-Iz)-Ixz^2)*q*r)/(Ix*Iz-Ixz^2);
qdot=(1/Iy)*(maero+p*r*(Iz-Ix)+Ixz*(r^2-p^2));
rdot=((Ixz*laero+Ix*naero)/(Ix*Iz-Ixz^2))+(((Ix*(Ix-Iy)+Ixz^2)*p*q-Ixz*(Ix-Iy+Iz)*q*r)/(Ix*Iz-Ixz^2));
%================================================
betadot=p*sin(alfa)-r*cos(alfa)+((M*g*cos(gama)*sin(mio))+(Y*cos(beta)-T*sin(beta)*cos(alfa)))/(M*V);
alfadot=q-(p*cos(alfa)+r*sin(alfa))*tan(beta)+(-L+M*g*cos(gama)*cos(mio)-T*sin(alfa))/(M*V*cos(beta));
miodot=1/cos(beta)*(p*cos(alfa)+r*sin(alfa))-g/V*tan(beta)*cos(mio)*cos(gama)+(L+T*sin(alfa))/(M*V)*(tan(gama)*sin(mio)+tan(beta))+Y/(M*V)*tan(gama)*cos(mio)*cos(beta);
%================================================
gamadot=((1/(M*V))*(-D*sin(beta)*sin(mio)+L*cos(mio)-M*g*cos(gama)-Y*sin(mio)*cos(beta)))+((T/(M*V))*(sin(mio)*sin(beta)*cos(alfa)+cos(mio)*sin(alfa)));
chidot=((L*sin(mio)+Y*cos(mio)*cos(beta))+T*(sin(mio)*sin(alfa)-cos(mio)*sin(beta)*cos(alfa)))/(M*V*cos(gama));
Vdot=(-D*cos(beta)+Y*sin(beta)-M*g*sin(gama)+T*cos(beta)*cos(alfa))/M;
%================================================
phidot=p+q*sin(phi)*tan(theta)+r*cos(phi)*tan(theta);
thetadot=q*cos(phi)-r*sin(phi);
psidot=(q*sin(phi)+r*cos(phi))/cos(theta);
%================================================
Dot=[pdot;qdot;rdot;betadot;alfadot;miodot;gamadot;chidot;Vdot;phidot;thetadot;psidot];

== matlab function nn+ekf/Kalman1 ==
  data: k1 output double; R1 output double; teta1 output double; P1 output double; k input double; R0 input double; teta0 input double; P0 input double; MM output double; yt input double; yT input double; M input double
function [k1,R1,teta1,P1,MM]  = fcn(k,R0,teta0,P0,yt,yT,M)
eta=1.5;
Z=teta0(2)*M+teta0(3)*yT;
sigma=(1-exp(-Z))/(1+exp(-Z));
H=[sigma;teta0(1)*M*0.5*(1-sigma^2);teta0(1)*yT*0.5*(1-sigma^2)];
R1=R0+(yt^2-R0)/k;
K=P0*H*(((H'*P0*H)+R1)^(-1));
teta1=teta0+eta*K*(yt);
n=teta1(2)*M+teta1(3)*yT;
MM=teta1(1)*((1-exp(-n))/(1+exp(-n)));
P1=P0-K*H'*P0;
k1=k+1;

== matlab function nn+ekf/Kalman2 ==
  data: k1 output double; R1 output double; teta1 output double; P1 output double; k input double; R0 input double; teta0 input double; P0 input double; MM output double; yt input double; yT input double; M input double
function [k1,R1,teta1,P1,MM]  = fcn(k,R0,teta0,P0,yt,yT,M)
eta=1;
Z=teta0(2)*M+teta0(3)*yT;
sigma=(1-exp(-Z))/(1+exp(-Z));
H=[sigma;teta0(1)*M*.5*(1-sigma^2);teta0(1)*yT*0.5*(1-sigma^2)];
R1=R0+(yt^2-R0)/k;
K=P0*H*(((H'*P0*H)+R1)^(-1));
teta1=teta0+eta*K*(yt);
n=teta1(2)*M+teta1(3)*yT;
MM=teta1(1)*((1-exp(-n))/(1+exp(-n)));
P1=P0-K*H'*P0;
k1=k+1;

== matlab function nn+ekf/Kalman3 ==
  data: k1 output double; R1 output double; teta1 output double; P1 output double; k input double; R0 input double; teta0 input double; P0 input double; MM output double; yt input double; yT input double; M input double
function [k1,R1,teta1,P1,MM] = fcn(k,R0,teta0,P0,yt,yT,M)
eta=1;
Z=teta0(2)*M+teta0(3)*yT;
sigma=(1-exp(-Z))/(1+exp(-Z));
H=[sigma;teta0(1)*M*0.5*(1-sigma^2);teta0(1)*yT*0.5*(1-sigma^2)];
R1=R0+(yt^2-R0)/k;
K=P0*H*(((H'*P0*H)+R1)^(-1));
teta1=teta0+eta*K*(yt);
n=teta1(2)*M+teta1(3)*yT;
MM=teta1(1)*((1-exp(-n))/(1+exp(-n)));
P1=P0-K*H'*P0;
k1=k+1;

== matlab function InnerLoop1/Inner loop Control ==
  data: beta input double; alfa input double; u output double; V input double; pqr input double; Uc input double; Upi input double
function u  = fcn(beta,alfa,V,pqr,Uc,Upi)

p=pqr(1);
q=pqr(2);
r=pqr(3);
%====================================
% Equations Of Motion
ro=.4139;%====================================================================================
cbar = 1.164; %======== m ========
c=cbar;
b = 25.83; %======== m ========
Ix = 2405;
Iy = 13987;
Iz = 14496;
Ixz = 909;
s = 27.8; %========= m^2 =======
Q=0.5*ro*V^2;
Clbeta=-0.0008569*180/pi; %per rad
Clp=-0.7417551; %per rad
Clr=0.1887752; %per rad
Cmq=-12.10793; %per rad
CldA=.0037483*180/pi; %per rad
CldR=.0006043*180/pi; %per rad
CmdE=-.0232702*180/pi; %per rad
Cnbeta=.0014660*180/pi; %per rad
Cnp=-0.0591078; %per rad
Cnr=-0.4654417; %per rad
CndA=.0000309*180/pi; %per rad
CndR=-.0010612*180/pi ; %per rad
Cm0= 0.0102;
Cmalfa=-1.31; % =========  1/rad =============
%===============================================
Cm =Cm0+cbar/(2*V)*Cmq*q;
%===============================================
L_aero=Q*s*b*(Clbeta*beta+(Clp*p+Clr*r)*b/(2*V));
M_aero=Q*s*c*(Cm0+Cmalfa*alfa+Cmq*q*c/(2*V));
N_aero=Q*s*b*(Cnbeta*beta+(Cnp*p+Cnr*r)*b/(2*V));

%==============================
f1=(Iz*L_aero+Ixz*N_aero+Ixz*(Ix-Iy+Iz)*p*q+(Iz*(Iy-Iz)-Ixz^2)*q*r)/(Ix*Iz-Ixz^2);
f2=(M_aero+p*r*(Iz-Ix)+Ixz*(r^2-p^2))/Iy;
f3=(Ixz*L_aero+Ix*N_aero+(Ix*(Ix-Iy)+Ixz^2)*p*q-Ixz*(Ix-Iy+Iz)*q*r)/(Ix*Iz-Ixz^2);


%==============================
LdA=(1/(Ix*Iz-Ixz^2))*(Q*s*b)*(Iz*CldA+Ixz*CndA);
LdR=(1/(Ix*Iz-Ixz^2))*(Q*s*b)*(Iz*CldR+Ixz*CndR);
MdE=(1/(Iy))*(Q*s*c)*CmdE;
NdA=(1/(Ix*Iz-Ixz^2))*(Q*s*b)*(Ix*CndA+Ixz*CldA);
NdR=(1/(Ix*Iz-Ixz^2))*(Q*s*b)*(Ix*CndR+Ixz*CldR);
%==============================
f_pqr=[f1;f2;f3];
B=([LdA 0 LdR;0 MdE 0;NdA 0 NdR]);
u=B\(Uc-f_pqr+Upi);

== matlab function InnerLoop1/PCH ==
  data: u input double; PCH output double; V input double
function PCH= fcn(u,V)


%====================================
% Equations Of Motion
ro=.4139;%====================================================================================
cbar = 1.164; %======== m ========
c=cbar;
b = 25.83; %======== m ========
Ix = 2405;
Iy = 13987;
Iz = 14496;
Ixz = 909;
s = 27.8; %========= m^2 =======
Q=0.5*ro*V^2;
Clbeta=-0.0008569*180/pi; %per rad
Clp=-0.7417551; %per rad
Clr=0.1887752; %per rad
Cmq=-12.10793; %per rad
CldA=.0037483*180/pi; %per rad
CldR=.0006043*180/pi; %per rad
CmdE=-.0232702*180/pi; %per rad
Cnbeta=.0014660*180/pi; %per rad
Cnp=-0.0591078; %per rad
Cnr=-0.4654417; %per rad
CndA=.0000309*180/pi; %per rad
CndR=-.0010612*180/pi ; %per rad
Cm0= 0.0102;
Cmalfa=-1.31; % =========  1/rad =============
%===============================================
LdA=(1/(Ix*Iz-Ixz^2))*(Q*s*b)*(Iz*CldA+Ixz*CndA);
LdR=(1/(Ix*Iz-Ixz^2))*(Q*s*b)*(Iz*CldR+Ixz*CndR);
MdE=(1/(Iy))*(Q*s*c)*CmdE;
NdA=(1/(Ix*Iz-Ixz^2))*(Q*s*b)*(Ix*CndA+Ixz*CldA);
NdR=(1/(Ix*Iz-Ixz^2))*(Q*s*b)*(Ix*CndR+Ixz*CldR);
%==============================
B=([LdA 0 LdR;0 MdE 0;NdA 0 NdR]);
PCH=B*u;

== matlab function Outer Loop1/Outer loop Control ==
  data: fbam output double; V input double; gs_inv output double; bam input double; pqr input double; dA input double; dE input double; dR input double; gama input double
function [fbam,gs_inv] = fcn(V,bam,pqr,dA,dE,dR,gama)
beta=bam(1);
alfa=bam(2);
mio=bam(3);
p=pqr(1);
q=pqr(2);
r=pqr(3);
% inputs ////////////////////
M = 5000; %=== mass  kg
th=1;
u0=140;%========================================================================================
ro=.4139;%====================================================================================
T = 13000*th*ro/1.225; %======== N ============
cbar = 1.164; %======== m ========
c=cbar;
b = 25.83; %======== m ========
s = 27.8; %========= m^2 =======
CLalfa=6.8; %per rad
CLq = 6.319133; %per rad
CLdE=.0054746*180/pi; %per rad
CLu=0;
Q=0.5*ro*V^2;
Cybeta=-0.0073848*180/pi; %per rad
Cyp=0.0367876; %per rad
Cyr=-1.5779230; %per rad
CydR=-.0050774*180/pi; %per rad
g = 9.81; %=== m/s^2 =====
CydA=.0001716*180/pi; %per rad
CL0=0.46;
%===============================================
Ybeta=Q*s*Cybeta/M;% (m/s^2)
Yp=Q*s*b*Cyp/(2*M*u0);% (m/s)
Yr=Q*s*b*Cyr/(2*M*u0);% (m/s)
YdR=Q*s*CydR/M; % (m/s^2)
YdA=Q*s*CydA/M; % (m/s^2)
%================================================
Y=M*(Ybeta*beta+Yp*p+Yr*r+YdR*dR+YdA*dA);
L=Q*s*(CL0+cbar/(2*V)*CLq*q+CLdE*dE);
%==============================
f1=(1/(M*V))*(Y*cos(beta)+M*g*sin(gama)*sin(mio)-T*sin(beta)*cos(alfa));
f2=(1/(M*V*cos(beta)))*(-L+M*g*cos(gama)*cos(mio)-T*sin(alfa));
f3=-g/V*tan(beta)*cos(mio)*cos(gama)+(1/(M*V))*((L+T*sin(alfa))*(tan(gama)*sin(mio)+tan(beta))+Y*tan(gama)*cos(mio)*cos(beta));
%==============================
fbam=[f1;f2;f3];
gs_inv=([sin(alfa) 0 -cos(alfa);-tan(beta)*cos(alfa) 1 -tan(beta)*sin(alfa);cos(alfa)/cos(beta) 0 sin(alfa)/cos(beta)])^-1;

== matlab function sensors additive  Fault 1 ==
  data: da input double; de input double; dr input double; fault output double; u input double; faulty_act output double
function [fault,faulty_act] = fcn(da,de,dr,u)
fault=[da;de;dr];
faulty_act=fault+u;
